simulink model "CEGR_TestBench_10kW_SimplifiedEGR_v01"  (R2025b)
settings: Solver=ode4  StartTime=0.0  StopTime=120  FixedStep=0.02  RelTol=1e-3
undefined symbols (not defined in the file): CaseBoundaryParam_simplified, CoolingCurveParam_simplified, dt_s_simplified, EGRInitialNode_simplified, PhysicalParam_simplified, StackInitialState_simplified, StackModelParam_simplified
settings Model: Creator=ADMIN  LastModifiedBy=ADMIN

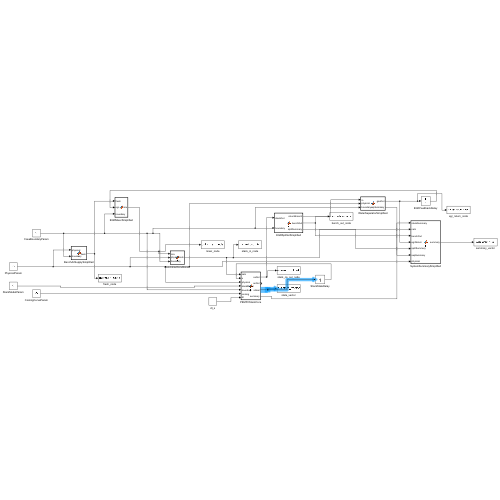
[thumbnail: Simulink's stored preview of the top-level diagram]
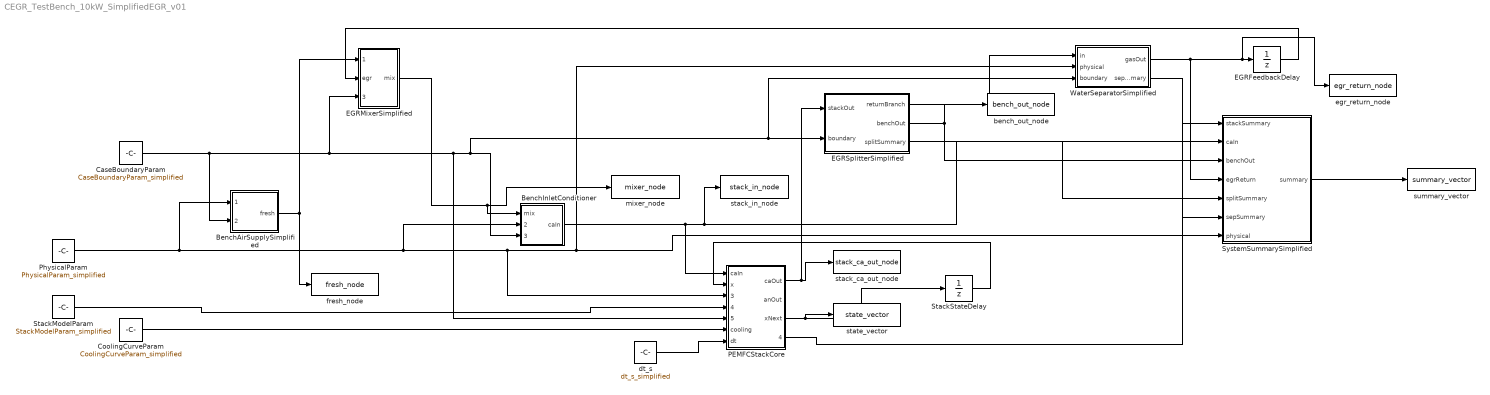
== system CEGR_TestBench_10kW_SimplifiedEGR_v01 ==
  BenchAirSupplySimplified : MATLAB Function  TreatAsAtomicUnit=on
  BenchInletConditioner : MATLAB Function  TreatAsAtomicUnit=on
  CaseBoundaryParam : Constant  Value=CaseBoundaryParam_simplified
  CoolingCurveParam : Constant  Value=CoolingCurveParam_simplified
  EGRFeedbackDelay : UnitDelay  InitialCondition=EGRInitialNode_simplified  SampleTime=dt_s_simplified
  EGRMixerSimplified : MATLAB Function  TreatAsAtomicUnit=on
  EGRSplitterSimplified : MATLAB Function  TreatAsAtomicUnit=on
  PEMFCStackCore : MATLAB Function  TreatAsAtomicUnit=on
  PhysicalParam : Constant  Value=PhysicalParam_simplified
  StackModelParam : Constant  Value=StackModelParam_simplified
  StackStateDelay : UnitDelay  InitialCondition=StackInitialState_simplified  SampleTime=dt_s_simplified
  SystemSummarySimplified : MATLAB Function  TreatAsAtomicUnit=on
  WaterSeparatorSimplified : MATLAB Function  TreatAsAtomicUnit=on
  bench_out_node : ToWorkspace  VariableName=bench_out_node  SaveFormat=Structure With Time
  dt_s : Constant  Value=dt_s_simplified
  egr_return_node : ToWorkspace  VariableName=egr_return_node  SaveFormat=Structure With Time
  fresh_node : ToWorkspace  VariableName=fresh_node  SaveFormat=Structure With Time
  mixer_node : ToWorkspace  VariableName=mixer_node  SaveFormat=Structure With Time
  stack_ca_out_node : ToWorkspace  VariableName=stack_ca_out_node  SaveFormat=Structure With Time
  stack_in_node : ToWorkspace  VariableName=stack_in_node  SaveFormat=Structure With Time
  state_vector : ToWorkspace  VariableName=state_vector  SaveFormat=Structure With Time
  summary_vector : ToWorkspace  VariableName=summary_vector  SaveFormat=Structure With Time
  wires:
  PhysicalParam/1 -> WaterSeparatorSimplified/2(physical), SystemSummarySimplified/7(physical), PEMFCStackCore/3(physical), BenchInletConditioner/2(physical), BenchAirSupplySimplified/1(physical)
  CaseBoundaryParam/1 -> PEMFCStackCore/5(boundary), EGRSplitterSimplified/2(boundary), WaterSeparatorSimplified/3(boundary), BenchInletConditioner/3(boundary), EGRMixerSimplified/3(boundary), BenchAirSupplySimplified/2(boundary)
  StackModelParam/1 -> PEMFCStackCore/4(stackModel)
  CoolingCurveParam/1 -> PEMFCStackCore/6(cooling)
  StackStateDelay/1 -> PEMFCStackCore/2(x)
  BenchAirSupplySimplified/1(fresh) -> EGRMixerSimplified/1(fresh), fresh_node/1
  EGRFeedbackDelay/1 -> EGRMixerSimplified/2(egr)
  EGRMixerSimplified/1(mix) -> mixer_node/1, BenchInletConditioner/1(mix)
  BenchInletConditioner/1(caIn) -> SystemSummarySimplified/2(caIn), stack_in_node/1, PEMFCStackCore/1(caIn)
  PEMFCStackCore/1(caOut) -> EGRSplitterSimplified/1(stackOut), stack_ca_out_node/1
  WaterSeparatorSimplified/1(gasOut) -> EGRFeedbackDelay/1, egr_return_node/1, SystemSummarySimplified/4(egrReturn)
  PEMFCStackCore/3(xNext) -> StackStateDelay/1, state_vector/1
  PEMFCStackCore/4(summary) -> SystemSummarySimplified/1(stackSummary)
  EGRSplitterSimplified/2(benchOut) -> bench_out_node/1, SystemSummarySimplified/3(benchOut)
  EGRSplitterSimplified/3(splitSummary) -> SystemSummarySimplified/5(splitSummary)
  WaterSeparatorSimplified/2(sepSummary) -> SystemSummarySimplified/6(sepSummary)
  SystemSummarySimplified/1(summary) -> summary_vector/1
  EGRSplitterSimplified/1(returnBranch) -> WaterSeparatorSimplified/1(in)
  dt_s/1 -> PEMFCStackCore/7(dt)

== matlab function CEGR_TestBench_10kW_SimplifiedEGR_v01/EGRMixerSimplified ==
  data: fresh input; mix output; egr input; boundary input
function mix = f(fresh, egr, boundary)
%#codegen
mTarget=max(boundary(4),1e-12); me0=max(sum(egr(1:3)),0); me=min(me0,0.95*mTarget); mf=max(mTarget-me,0);
wf=fresh(1:4)/max(sum(fresh(1:4)),1e-12); we=egr(1:4)/max(sum(egr(1:4)),1e-12);
mix=zeros(7,1); mix(1:4)=mf*wf+me*we; mt=max(mf+me,1e-12);
mix(5)=(fresh(5)*mf+egr(5)*me)/mt; mix(6)=fresh(6); mix(7)=double(mix(4)>1e-12);
end

== matlab function CEGR_TestBench_10kW_SimplifiedEGR_v01/BenchAirSupplySimplified ==
  data: physical input; fresh output; boundary input
function fresh = f(physical, boundary)
%#codegen
wO2=max(boundary(5),0); wN2=max(boundary(6),0); wV=max(boundary(7),0); s=max(wO2+wN2+wV,1e-12);
fresh=[wO2/s; wN2/s; wV/s; 0; boundary(3); boundary(2); 0];
end

== matlab function CEGR_TestBench_10kW_SimplifiedEGR_v01/BenchInletConditioner ==
  data: mix input; caIn output; physical input; boundary input
function caIn = f(mix, physical, boundary)
%#codegen
M_O2=physical(3); M_N2=physical(4); M_H2O=physical(5); p=boundary(2); T=boundary(3);
caIn=mix; caIn(5)=T; caIn(6)=p;
ps=min(sat_kPa(T),0.98*p); nDry=max(caIn(1)/M_O2+caIn(2)/M_N2,1e-12); mSat=ps*nDry/max(p-ps,1e-6)*M_H2O;
if caIn(3)>mSat, caIn(4)=caIn(4)+caIn(3)-mSat; caIn(3)=mSat; end
caIn(7)=double(caIn(4)>1e-12);
end
function p=sat_kPa(T)
Tc=min(max(T,-40),120); p=0.61121*exp((18.678-Tc/234.5)*(Tc/(257.14+Tc)));
end

== matlab function CEGR_TestBench_10kW_SimplifiedEGR_v01/PEMFCStackCore ==
  data: caIn input; caOut output; x input; physical input; stackModel input; anOut output; xNext output; summary output; boundary input; cooling input; dt input
function [caOut, anOut, xNext, summary] = f(caIn, x, physical, stackModel, boundary, cooling, dt)
%#codegen
R=physical(1); F=physical(2); M_O2=physical(3); M_N2=physical(4); M_H2O=physical(5); M_H2=physical(6); pamb=physical(7); Tamb=physical(8);
N=stackModel(1); A=stackModel(2); Vca=stackModel(3); Van=stackModel(4); Kca=stackModel(5); Kan=stackModel(6); Cfc=stackModel(7); hCool=stackModel(8); hAmb=stackModel(9);
Eref=stackModel(10); Etemp=stackModel(11); th1=stackModel(12); th2=stackModel(13); th3=stackModel(14); th4=stackModel(15); deltaCm=stackModel(16); th8=stackModel(17); th9=stackModel(18); th10=stackModel(19); Vtn=stackModel(20); th5=stackModel(21); th6=stackModel(22); th7=stackModel(23); tauMem=stackModel(24);
I=boundary(1); pcBack=boundary(8); anFlow=boundary(12); anWH2=boundary(13); anWV=boundary(14); panBack=boundary(15); Tcool=boundary(16); coolantFlow=boundary(17);
hCoolEff=hCool; nCool=floor((numel(cooling)-1)/2); if nCool>=2 && cooling(1)>0.5, hCoolEff=interp_hcool_flow(coolantFlow,cooling(2:1+nCool),cooling(2+nCool:1+2*nCool),hCool); end
mO2=max(x(1),1e-12); mN2=max(x(2),1e-12); mV=max(x(3),0); mH2=max(x(4),1e-12); mVAn=max(x(5),0); T=x(6); TK=T+273.15; mMemPrev=0; if numel(x)>=7, mMemPrev=x(7); end
pO2=mO2/M_O2*R*TK/Vca/1000; pN2=mN2/M_N2*R*TK/Vca/1000; pV=mV/M_H2O*R*TK/Vca/1000; pCa=max(pO2+pN2+pV,pamb); pVAn=mVAn/M_H2O*R*TK/Van/1000;
mInCmd=sum(caIn(1:3)); mIn=mInCmd; wIn=caIn(1:3)/max(mInCmd,1e-12); mO2In=mIn*wIn(1); mN2In=mIn*wIn(2); mVIn=mIn*wIn(3);
mO2React=I*N/(4*F)*M_O2; mH2React=I*N/(2*F)*M_H2; mWater=I*N/(2*F)*M_H2O; lambdaO2=(mO2In/M_O2)/max(I*N/(4*F),1e-12);
ps=sat_kPa(T); aCa=min(max(pV/max(ps,1e-6),0),3); aAn=min(max(pVAn/max(ps,1e-6),0),3); lambdaCa=lambda_eq(aCa); lambdaAn=lambda_eq(aAn); lam=0.5*(lambdaCa+lambdaAn);
mH2In=max(anFlow,0)*min(max(anWH2,0),1); mVAnIn=max(anFlow,0)*min(max(anWV,0),1);
A_m2=A*1e-4; delta_m=max(deltaCm*0.01,1e-9); nDrag=max(0.0029*lam^2+0.05*lam,0); D=membrane_diff(lam,TK); rhoMem=2000; EW=1.10; cMemCa=rhoMem/EW*lambdaCa; cMemAn=rhoMem/EW*lambdaAn; JDrag=nDrag*I/(F*max(A_m2,1e-12)); JDiff=D/max(delta_m,1e-12)*(cMemCa-cMemAn); JNetRaw=JDrag-JDiff; nDragMol=JDrag*A_m2*N; nDiffMol=JDiff*A_m2*N; mDrag=JDrag*A_m2*N*M_H2O; mDiff=JDiff*A_m2*N*M_H2O; mMemRaw=JNetRaw*A_m2*N*M_H2O; mMemMaxPos=max(mVAn+dt*mVAnIn,0)/max(dt,1e-9); mMemMaxNeg=-max(mV+dt*(mVIn+mWater),0)/max(dt,1e-9); mMemTarget=min(max(mMemRaw,mMemMaxNeg),mMemMaxPos); alpha=min(max(dt/max(tauMem,dt),0),1); mMemRelax=mMemPrev+alpha*(mMemTarget-mMemPrev); mMem=min(max(mMemRelax,mMemMaxNeg),mMemMaxPos); JNet=mMem/max(A_m2*N*M_H2O,1e-18); mMemLimit=mMem-mMemRaw;
mO2Pre=max(mO2+dt*(mO2In-mO2React),1e-12); mN2Pre=max(mN2+dt*mN2In,1e-12); mVPre=max(mV+dt*(mVIn+mWater+mMem),0); mH2Pre=max(mH2+dt*(mH2In-mH2React),1e-12); mVAnPre=max(mVAn+dt*(mVAnIn-mMem),0);
pO2Pre=mO2Pre/M_O2*R*TK/Vca/1000; pN2Pre=mN2Pre/M_N2*R*TK/Vca/1000; pVPre=mVPre/M_H2O*R*TK/Vca/1000; pCaPre=max(pO2Pre+pN2Pre+pVPre,pamb); pH2Pre=mH2Pre/M_H2*R*TK/Van/1000; pVAnPre=mVAnPre/M_H2O*R*TK/Van/1000; pAnPre=max(pH2Pre+pVAnPre,pamb);
gasCa=max(mO2Pre+mN2Pre+mVPre,1e-12); wO2=mO2Pre/gasCa; wN2=mN2Pre/gasCa; wV=mVPre/gasCa; mCaOutRaw=Kca*max(pCaPre-pcBack,0)/(1+Kca*max(pCaPre,1e-6)*dt/gasCa); mCaOut=min(mCaOutRaw,0.95*gasCa/max(dt,1e-9));
gasAn=max(mH2Pre+mVAnPre,1e-12); wH2=mH2Pre/gasAn; wVAn=mVAnPre/gasAn; mAnOutRaw=Kan*max(pAnPre-panBack,0)/(1+Kan*max(pAnPre,1e-6)*dt/gasAn); mAnOut=min(mAnOutRaw,0.95*gasAn/max(dt,1e-9));
mO2n=max(mO2Pre-dt*wO2*mCaOut,1e-12); mN2n=max(mN2Pre-dt*wN2*mCaOut,1e-12); mVnRaw=max(mVPre-dt*wV*mCaOut,0); mH2n=max(mH2Pre-dt*wH2*mAnOut,1e-12); mVAnnRaw=max(mVAnPre-dt*wVAn*mAnOut,0);
j=max(I/max(A,1e-9),1e-6); E=Eref-Etemp*(TK-298.15)+R*TK/(2*F)*log(max(pH2Pre*1000,1)/101325*sqrt(max(pO2Pre*1000,1)/101325)); CO2=max(1.97e-7*(pO2Pre*1000)*exp(498/TK),1e-12); etaAct=max(th1+th2*TK+th3*TK*log(CO2)+th4*TK*log(max(I,1e-6)),0); Rm=deltaCm/max(A*(th5*lam+th6)*exp(th7*(1/303.15-1/TK)),1e-12); etaOhm=I*(Rm+th8); iLim=j; i0Scale=CO2; etaCon=max(th9*exp(min(th10*I,50)),0);
V=E-etaAct-etaOhm-etaCon; Pstack=I*V*N; Qgen=I*N*(Vtn-V); Qcool=hCoolEff*(T-Tcool); Qamb=hAmb*(T-Tamb); Qgas=max(mCaOut+mAnOut,0)*1050*max(T-caIn(5),0); Qnet=Qgen-Qcool-Qamb-Qgas; Tn=T+dt*Qnet/Cfc;
[mVn,liqDiag,psCaNext]=clip_vapor_inventory(mVnRaw,Vca,Tn,physical); [mVAnn,liqAnDiag,psAnNext]=clip_vapor_inventory(mVAnnRaw,Van,Tn,physical); phaseCa=(mVnRaw-mVn)/dt; phaseAn=(mVAnnRaw-mVAnn)/dt;
TKn=Tn+273.15; pO2Diag=mO2n/M_O2*R*TKn/Vca/1000; pN2Diag=mN2n/M_N2*R*TKn/Vca/1000; pVDiag=mVn/M_H2O*R*TKn/Vca/1000; pCaDiag=max(pO2Diag+pN2Diag+pVDiag,pamb); pH2Diag=mH2n/M_H2*R*TKn/Van/1000; pVAnDiag=mVAnn/M_H2O*R*TKn/Van/1000; pAnDiag=max(pH2Diag+pVAnDiag,pamb);
xNext=[mO2n;mN2n;mVn;mH2n;mVAnn;Tn;mMem]; caOut=[wO2*mCaOut;wN2*mCaOut;wV*mCaOut;0;Tn+3;pcBack;0]; anOut=[wH2*mAnOut;0;wVAn*mAnOut;0;Tn;panBack;0];
nTot=max(mO2n/M_O2+mN2n/M_N2+mVn/M_H2O,1e-12); xO2=(mO2n/M_O2)/nTot; RH=pVDiag/max(sat_kPa(Tn),1e-6); nInTot=max(caIn(1)/M_O2+caIn(2)/M_N2+caIn(3)/M_H2O,1e-12); xO2In=(caIn(1)/M_O2)/nInTot; pO2In=caIn(6)*xO2In; RHIn=(caIn(6)*(caIn(3)/M_H2O)/nInTot)/max(sat_kPa(caIn(5)),1e-6);
resO2=(mO2n-mO2)/dt-(mO2In-wO2*mCaOut-mO2React); resN2=(mN2n-mN2)/dt-(mN2In-wN2*mCaOut); resH2Ov=(mVn-mV)/dt-(mVIn-wV*mCaOut+mWater+mMem-phaseCa); resH2=(mH2n-mH2)/dt-(mH2In-wH2*mAnOut-mH2React); resH2OvAn=(mVAnn-mVAn)/dt-(mVAnIn-wVAn*mAnOut-mMem-phaseAn); maxGasRes=max(abs([resO2,resN2,resH2Ov,resH2,resH2OvAn]));
summary=[I;V;Pstack;pO2Diag;pCaDiag;pH2Diag;pAnDiag;lam;Tn;xO2;RH;mMem;mO2React;mH2React;mWater;mCaOut;mAnOut;Cfc*(Tn-T)/dt-Qnet;pO2In;xO2In;RHIn;Qnet;resO2;resN2;resH2Ov;phaseCa;resH2;resH2OvAn;phaseAn;phaseCa+phaseAn;maxGasRes;Qgen;Qcool;Qamb;Qgas;E;etaAct;etaOhm;etaCon;lambdaO2;mIn;iLim;i0Scale;mVIn;wV*mCaOut;mVAnIn;wVAn*mAnOut;liqDiag+liqAnDiag;lambdaCa;lambdaAn;nDragMol;nDiffMol;psCaNext;psAnNext;mVnRaw;mVAnnRaw;liqDiag;liqAnDiag;JDrag;JDiff;JNet;mDrag;mDiff;mMemRaw;mMemLimit;mMemTarget;tauMem];
end
function [mv,condensed,ps]=clip_vapor_inventory(mv0,V,T,physical)
R=physical(1); M_H2O=physical(5); TK=T+273.15; ps=sat_kPa(T); mSat=max(ps*1000*V*M_H2O/(R*TK),0); if mv0>mSat, mv=mSat; condensed=mv0-mSat; else, mv=mv0; condensed=0; end
end
function p=sat_kPa(T)
Tc=min(max(T,-40),120); p=0.61121*exp((18.678-Tc/234.5)*(Tc/(257.14+Tc)));
end
function lambda=lambda_eq(a)
if a<=1, lambda=0.043+17.81*a-39.85*a^2+36*a^3; else, lambda=14+1.4*(a-1); end
end
function D=membrane_diff(lambda,TK)
if lambda<2, d0=1e-10; elseif lambda<3, d0=1e-10*(1+2*(lambda-2)); elseif lambda<4.5, d0=1e-10*(3-1.167*(lambda-3)); else, d0=1.25e-10; end; D=d0*exp(2416*(1/303-1/max(TK,1)));
end
function h=interp_hcool_flow(flow,bp,hv,hFallback)
n=0; for k=1:numel(bp), if bp(k)>0 && hv(k)>0, n=n+1; end, end; if n<2, h=hFallback; return; end; b=zeros(n,1); v=zeros(n,1); j=0; for k=1:numel(bp), if bp(k)>0 && hv(k)>0, j=j+1; b(j)=bp(k); v(j)=hv(k); end, end; if flow<=b(1), h=v(1); return; end; if flow>=b(n), h=v(n); return; end; h=v(n); for k=1:n-1, if flow>=b(k) && flow<=b(k+1), a=(flow-b(k))/max(b(k+1)-b(k),1e-9); h=v(k)+a*(v(k+1)-v(k)); return; end, end
end

== matlab function CEGR_TestBench_10kW_SimplifiedEGR_v01/EGRSplitterSimplified ==
  data: stackOut input; returnBranch output; boundary input; benchOut output; splitSummary output
function [returnBranch, benchOut, splitSummary] = f(stackOut, boundary)
%#codegen
r=min(max(boundary(11),0),0.95); returnBranch=stackOut; returnBranch(1:4)=r*stackOut(1:4); returnBranch(7)=double(returnBranch(4)>1e-12);
benchOut=stackOut; benchOut(1:4)=(1-r)*stackOut(1:4); benchOut(7)=double(benchOut(4)>1e-12);
mOutGas=sum(stackOut(1:3)); splitSummary=[r;sum(returnBranch(1:3));sum(benchOut(1:3));mOutGas;stackOut(4);returnBranch(4);benchOut(4)];
end

== matlab function CEGR_TestBench_10kW_SimplifiedEGR_v01/WaterSeparatorSimplified ==
  data: in input; gasOut output; physical input; sepSummary output; boundary input
function [gasOut, sepSummary] = f(in, physical, boundary)
%#codegen
M_O2=physical(3); M_N2=physical(4); M_H2O=physical(5); gasOut=in; gasOut(5)=boundary(9); gasOut(6)=boundary(10);
p=max(gasOut(6),1e-6); T=gasOut(5); ps=min(sat_kPa(T),0.98*p); nDry=max(gasOut(1)/M_O2+gasOut(2)/M_N2,1e-12); mSat=ps*nDry/max(p-ps,1e-6)*M_H2O;
condensed=max(gasOut(3)-mSat,0); gasOut(3)=gasOut(3)-condensed; drain=gasOut(4)+condensed; gasOut(4)=0; gasOut(7)=0;
sepSummary=[drain;condensed;in(4);rel_hum(gasOut,M_O2,M_N2,M_H2O);T;p;sum(gasOut(1:3))];
end
function rh=rel_hum(node,M_O2,M_N2,M_H2O)
nV=max(node(3)/M_H2O,0); nt=max(node(1)/M_O2+node(2)/M_N2+nV,1e-12); rh=node(6)*nV/nt/max(sat_kPa(node(5)),1e-6);
end
function p=sat_kPa(T)
Tc=min(max(T,-40),120); p=0.61121*exp((18.678-Tc/234.5)*(Tc/(257.14+Tc)));
end

== matlab function CEGR_TestBench_10kW_SimplifiedEGR_v01/SystemSummarySimplified ==
  data: stackSummary input; summary output; caIn input; benchOut input; egrReturn input; splitSummary input; sepSummary input; physical input
function summary = f(stackSummary, caIn, benchOut, egrReturn, splitSummary, sepSummary, physical)
%#codegen
M_O2=physical(3); M_N2=physical(4); M_H2O=physical(5); nIn=max(caIn(1)/M_O2+caIn(2)/M_N2+caIn(3)/M_H2O,1e-12);
xO2In=(caIn(1)/M_O2)/nIn; mIn=sum(caIn(1:3)); mEgr=sum(egrReturn(1:3)); mBenchOut=sum(benchOut(1:3));
summary=[stackSummary; xO2In; mIn; mEgr; mBenchOut; splitSummary; sepSummary];
end
